simulink model "sim2_control_Architectures"  (R2022a)
settings: Solver=FixedStepAuto  StartTime=0.0  StopTime=8  FixedStep=0.001  RelTol=1e-3
undefined symbols (not defined in the file): a, b, c, DiscIntNeverNeededParam, k1, k2, kd2, kd3, kd4, ki3, kp1, kp2, kp3, kp4
libraries: slpidlib x2
settings Model: Creator=sokserey  LastModifiedBy=LabPC
settings DebuggingCC: UnconnectedInputMsg=warning  UnconnectedOutputMsg=warning  UnconnectedLineMsg=warning
settings RTWCC: DLArmComputeVersion=19.05

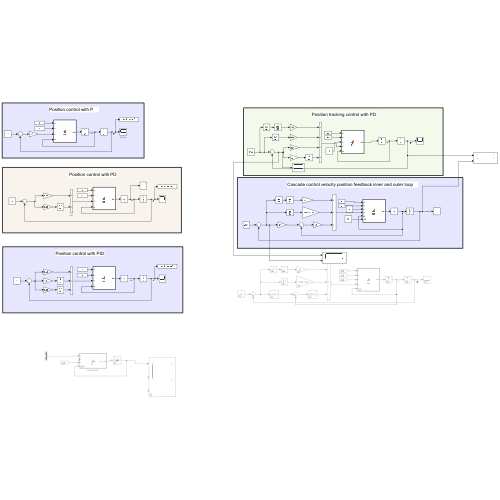
[thumbnail: Simulink's stored preview of the top-level diagram]
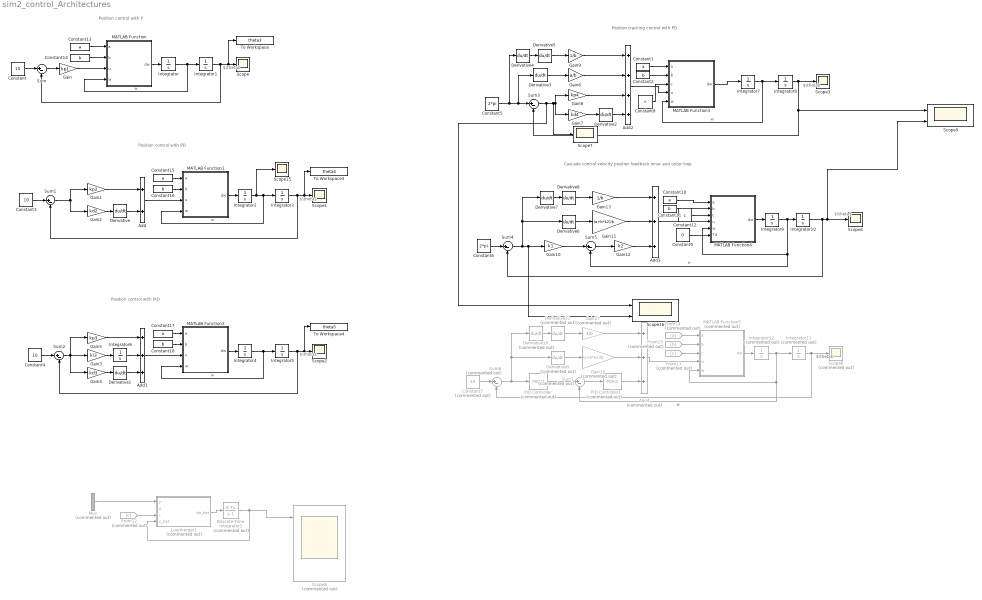
== system sim2_control_Architectures ==
  note: Position control with P
  note: Position control with PD
  note: $\theta$
  note: $\theta$
  note: $\theta$
  note: Position control with PID
  note: $\theta$
  note: Position tracking control with PD
  note: $\theta$
  note: Cascade control velocity position feedback inner and outer loop
  note: $\theta$
  Add : Sum
  Add1 : Sum  Inputs=+++
  Add2 : Sum  Inputs=++++
  Add3 : Sum  Inputs=+++
  Add4 : Sum  Commented=on  Inputs=+++
  Constant : Constant  Value=10
  Constant{1,10,13,15,17} (5 alike) : Constant  Value=a
  Constant{2,11,14,16,18} (5 alike) : Constant  Value=b
  Constant12 : Constant  Value=c
  Constant3 : Constant  Value=10
  Constant4 : Constant  Value=10
  Constant5 : Constant  Value=2*pi
  Constant6 : Constant  Value=2*pi
  Constant7 : Constant  Commented=on  Value=10
  Constant8 : Constant  Value=c
  Constant9 : Constant  Value=0
  Derivative{,1..8} (9 alike) : Derivative
  Derivative10 : Derivative  Commented=on
  Derivative11 : Derivative  Commented=on
  Derivative9 : Derivative  Commented=on
  Discrete-Time Integrator2 : DiscreteIntegrator  Commented=on  InitialCondition=[0;0]  SampleTime=0.01  ICPrevOutput=DiscIntNeverNeededParam  ICPrevScaledInput=DiscIntNeverNeededParam
  From12 : From  Commented=on  GotoTag=c
  From13 : From  Commented=on  GotoTag=c
  From14 : From  Commented=on  GotoTag=a
  From15 : From  Commented=on  GotoTag=b
  Gain : Gain  Gain=kp1
  Gain1 : Gain  Gain=kp2
  Gain10 : Gain  Gain=k1
  Gain11 : Gain  Gain=(a+b*k2)/b
  Gain12 : Gain  Gain=k2
  Gain13 : Gain  Gain=1/b
  Gain15 : Gain  Commented=on  Gain=(a+b*k2)/b
  Gain17 : Gain  Commented=on  Gain=1/b
  Gain2 : Gain  Gain=kd2
  Gain3 : Gain  Gain=ki3
  Gain4 : Gain  Gain=kd3
  Gain5 : Gain  Gain=kp3
  Gain6 : Gain  Gain=kp4
  Gain7 : Gain  Gain=kd4
  Gain8 : Gain  Gain=a/b
  Gain9 : Gain  Gain=1/b
  Integrator{,1..10} (11 alike) : Integrator
  Integrator11 : Integrator  Commented=on
  Integrator12 : Integrator  Commented=on
  Luenberger1 : MATLAB Function  Commented=on  TreatAsAtomicUnit=on
  MATLAB Function : MATLAB Function  TreatAsAtomicUnit=on
  MATLAB Function1 : MATLAB Function  TreatAsAtomicUnit=on
  MATLAB Function2 : MATLAB Function  TreatAsAtomicUnit=on
  MATLAB Function3 : MATLAB Function  TreatAsAtomicUnit=on
  MATLAB Function4 : MATLAB Function  TreatAsAtomicUnit=on
  MATLAB Function5 : MATLAB Function  Commented=on  TreatAsAtomicUnit=on
  Mux : Mux  Commented=on  Inputs=2
  PID Controller : slpidlib/PID Controller  Commented=on  Controller=PID  Form=Parallel  TimeDomain=Discrete-time  UseExternalTs=off  SampleTime=-1  IntegratorMethod=Forward Euler  FilterMethod=Forward Euler  ControllerParametersSource=internal  P=0.000211921225364968  I=9.98226441094489e-09  UseKiTs=off  D=0.999605299326111  N=0.722686382801031  UseFilter=on  TunerSelectOption=Transfer Function Based (PID Tuner App)  InitialConditionSource=internal  InitialConditionForIntegrator=0  InitialConditionForFilter=0  DifferentiatorICPrevScaledInput=0  ExternalReset=none  TrackingMode=off  Kt=1  LimitOutput=off  SatLimitsSource=internal  UpperSaturationLimit=inf  LowerSaturationLimit=-inf  LinearizeAsGain=on  AntiWindupMode=none  Kb=1  POutMin=[]  POutMax=[]  IOutMin=[]  IOutMax=[]  DOutMin=[]  DOutMax=[]  NOutMin=[]  NOutMax=[]  SumOutMin=[]  SumOutMax=[]  SaturationOutMin=[]  SaturationOutMax=[]  PParamMin=[]  PParamMax=[]  IParamMin=[]  IParamMax=[]  DParamMin=[]  DParamMax=[]  NParamMin=[]  NParamMax=[]  KbParamMin=[]  KbParamMax=[]  KtParamMin=[]  KtParamMax=[]  KbOutMin=[]  KbOutMax=[]  KtOutMin=[]  KtOutMax=[]  IntegratorOutMin=[]  IntegratorOutMax=[]  FilterOutMin=[]  FilterOutMax=[]  SumI1OutMin=[]  SumI1OutMax=[]  SumI2OutMin=[]  SumI2OutMax=[]  SumI3OutMin=[]  SumI3OutMax=[]  SumI4OutMin=[]  SumI4OutMax=[]  SumDOutMin=[]  SumDOutMax=[]  DifferentiatorOutMin=[]  DifferentiatorOutMax=[]  FilterDiffOutCoefMin=[]  FilterDiffOutCoefMax=[]  ReciprocalOutMin=[]  ReciprocalOutMax=[]  SumDenOutMin=[]  SumDenOutMax=[]  SumNumOutMin=[]  SumNumOutMax=[]  DivideOutMin=[]  DivideOutMax=[]  UdiffTsProdOutMin=[]  UdiffTsProdOutMax=[]  NTsProdOutMin=[]  NTsProdOutMax=[]  UintegralTsProdOutMin=[]  UintegralTsProdOutMax=[]  UngainTsProdOutMin=[]  UngainTsProdOutMax=[]  IntegratorContinuousStateAttributes=''  IntegratorStateMustResolveToSignalObject=off  IntegratorRTWStateStorageClass=Auto  FilterContinuousStateAttributes=''  FilterStateMustResolveToSignalObject=off  FilterRTWStateStorageClass=Auto  ParallelPVariant=InternalParameters  IdealPVariant=Disabled  IVariant=InternalParameters  DVariant=InternalParameters  IntegratorVariant=Discrete  SatVariant=Disabled  AWVariant=Passthrough  PCopyVariant=Disabled  TRVariant=Disabled  FdbkBlocksVariant=Forward  IdealPFdbkVariant=Disabled  SatFdbkVariant=Disabled  DerivativeFilterVariant=ForwardEulerFilter  NVariant=InternalParameters  NCopyVariant=Disabled  FilterICVariant=InternalICsFilter  IntegratorICVariant=InternalICs  ExternalResetVariant=Disabled  TRSumVariant=Passthrough  SumFdbkVariant=Disabled  SumVariant=Sum_PID  TsampFilterVariant=InternalTs  TsampNgainVariant=Passthrough  TsampIntegralVariant=Passthrough  ExternalSaturationOutDataTypeStr=Inherit: Same as second input  aMode=0
  PID Controller1 : slpidlib/PID Controller  Commented=on  Controller=PID  Form=Parallel  TimeDomain=Discrete-time  UseExternalTs=off  SampleTime=-1  IntegratorMethod=Forward Euler  FilterMethod=Forward Euler  ControllerParametersSource=internal  P=0.27  I=1  UseKiTs=off  D=0  N=100  UseFilter=on  TunerSelectOption=Transfer Function Based (PID Tuner App)  InitialConditionSource=internal  InitialConditionForIntegrator=0  InitialConditionForFilter=0  DifferentiatorICPrevScaledInput=0  ExternalReset=none  TrackingMode=off  Kt=1  LimitOutput=off  SatLimitsSource=internal  UpperSaturationLimit=inf  LowerSaturationLimit=-inf  LinearizeAsGain=on  AntiWindupMode=none  Kb=1  POutMin=[]  POutMax=[]  IOutMin=[]  IOutMax=[]  DOutMin=[]  DOutMax=[]  NOutMin=[]  NOutMax=[]  SumOutMin=[]  SumOutMax=[]  SaturationOutMin=[]  SaturationOutMax=[]  PParamMin=[]  PParamMax=[]  IParamMin=[]  IParamMax=[]  DParamMin=[]  DParamMax=[]  NParamMin=[]  NParamMax=[]  KbParamMin=[]  KbParamMax=[]  KtParamMin=[]  KtParamMax=[]  KbOutMin=[]  KbOutMax=[]  KtOutMin=[]  KtOutMax=[]  IntegratorOutMin=[]  IntegratorOutMax=[]  FilterOutMin=[]  FilterOutMax=[]  SumI1OutMin=[]  SumI1OutMax=[]  SumI2OutMin=[]  SumI2OutMax=[]  SumI3OutMin=[]  SumI3OutMax=[]  SumI4OutMin=[]  SumI4OutMax=[]  SumDOutMin=[]  SumDOutMax=[]  DifferentiatorOutMin=[]  DifferentiatorOutMax=[]  FilterDiffOutCoefMin=[]  FilterDiffOutCoefMax=[]  ReciprocalOutMin=[]  ReciprocalOutMax=[]  SumDenOutMin=[]  SumDenOutMax=[]  SumNumOutMin=[]  SumNumOutMax=[]  DivideOutMin=[]  DivideOutMax=[]  UdiffTsProdOutMin=[]  UdiffTsProdOutMax=[]  NTsProdOutMin=[]  NTsProdOutMax=[]  UintegralTsProdOutMin=[]  UintegralTsProdOutMax=[]  UngainTsProdOutMin=[]  UngainTsProdOutMax=[]  IntegratorContinuousStateAttributes=''  IntegratorStateMustResolveToSignalObject=off  IntegratorRTWStateStorageClass=Auto  FilterContinuousStateAttributes=''  FilterStateMustResolveToSignalObject=off  FilterRTWStateStorageClass=Auto  ParallelPVariant=InternalParameters  IdealPVariant=Disabled  IVariant=InternalParameters  DVariant=InternalParameters  IntegratorVariant=Discrete  SatVariant=Disabled  AWVariant=Passthrough  PCopyVariant=Disabled  TRVariant=Disabled  FdbkBlocksVariant=Forward  IdealPFdbkVariant=Disabled  SatFdbkVariant=Disabled  DerivativeFilterVariant=ForwardEulerFilter  NVariant=InternalParameters  NCopyVariant=Disabled  FilterICVariant=InternalICsFilter  IntegratorICVariant=InternalICs  ExternalResetVariant=Disabled  TRSumVariant=Passthrough  SumFdbkVariant=Disabled  SumVariant=Sum_PID  TsampFilterVariant=InternalTs  TsampNgainVariant=Passthrough  TsampIntegralVariant=Passthrough  ExternalSaturationOutDataTypeStr=Inherit: Same as second input  aMode=0
  Scope{,1..4,7,15} (7 alike) : Scope
  Scope16 : Scope  NumInputPorts=2
  Scope5 : Scope  NumInputPorts=2
  Scope6 : Scope  Commented=on
  Scope8 : Scope  Commented=on  NumInputPorts=3
  Sum{,1..5} (6 alike) : Sum  Inputs=|+-
  Sum6 : Sum  Commented=on  Inputs=|+-
  Sum7 : Sum  Commented=on  Inputs=|+-
  To Workspace : ToWorkspace  VariableName=theta3  SampleTime=-1
      settings: Save2DSignal=2-D array (concatenate along first dimension)
  To Workspace3 : ToWorkspace  VariableName=theta4  SampleTime=-1
      settings: Save2DSignal=2-D array (concatenate along first dimension)
  To Workspace4 : ToWorkspace  VariableName=theta5  SampleTime=-1
      settings: Save2DSignal=2-D array (concatenate along first dimension)
  wires:
  Gain/1 -> MATLAB Function/3(u)
  Sum2/1 -> Gain4/1, Gain5/1, Gain3/1
  Constant16/1 -> MATLAB Function1/2(b)
  Add1/1 -> MATLAB Function2/3(u)
  Integrator1/1 -> Sum/2, To Workspace/1, Scope/1
  Sum/1 -> Gain/1
  Gain5/1 -> Add1/1
  Constant4/1 -> Sum2/1
  Gain1/1 -> Add/1
  MATLAB Function2/1(dw) -> Integrator4/1
  Constant15/1 -> MATLAB Function1/1(a)
  Constant3/1 -> Sum1/1
  Gain4/1 -> Derivative1/1
  Derivative/1 -> Add/2
  Integrator5/1 -> Sum2/2, Scope2/1, To Workspace4/1
  Add/1 -> MATLAB Function1/3(u)
  Integrator2/1 -> Scope15/1, MATLAB Function1/4(w), Integrator3/1  "w"
  Integrator/1 -> Integrator1/1, MATLAB Function/4(w)  "w"
  Integrator4/1 -> Integrator5/1, MATLAB Function2/4(w)  "w"
  Constant18/1 -> MATLAB Function2/2(b)
  Sum1/1 -> Gain2/1, Gain1/1
  Constant17/1 -> MATLAB Function2/1(a)
  Gain2/1 -> Derivative/1
  Gain3/1 -> Integrator6/1
  Integrator3/1 -> To Workspace3/1, Scope1/1, Sum1/2
  Constant/1 -> Sum/1
  MATLAB Function/1(dw) -> Integrator/1
  Derivative1/1 -> Add1/3
  MATLAB Function1/1(dw) -> Integrator2/1
  Integrator6/1 -> Add1/2
  Integrator8/1 -> Scope5/1, Sum3/2, Scope3/1
  Gain7/1 -> Derivative2/1
  Sum3/1 -> Scope16/1, Scope7/1, Gain6/1, Gain7/1
  Integrator7/1 -> Integrator8/1, MATLAB Function3/5(w)  "w"
  Add2/1 -> MATLAB Function3/4(u)
  Constant5/1 -> Derivative4/1, Derivative3/1, Sum3/1
  Constant1/1 -> MATLAB Function3/1(a)
  Constant2/1 -> MATLAB Function3/2(b)
  Gain9/1 -> Add2/1
  Gain8/1 -> Add2/2
  Gain6/1 -> Add2/3
  Derivative2/1 -> Add2/4
  MATLAB Function3/1(dw) -> Integrator7/1
  Derivative3/1 -> Gain8/1
  Derivative4/1 -> Derivative5/1
  Derivative5/1 -> Gain9/1
  MATLAB Function4/1(dw) -> Integrator9/1
  Integrator10/1 -> Scope5/2, Scope4/1, Sum4/2
  Sum4/1 -> Derivative6/1, Derivative7/1, Scope16/2, Gain10/1
  Integrator9/1 -> Integrator10/1, MATLAB Function4/5(w), Sum5/2  "w"
  Constant6/1 -> Sum4/1
  Gain10/1 -> Sum5/1
  Sum5/1 -> Gain12/1
  Gain12/1 -> Add3/3
  Gain11/1 -> Add3/2
  Gain13/1 -> Add3/1
  Derivative7/1 -> Derivative8/1
  Derivative8/1 -> Gain13/1
  Derivative6/1 -> Gain11/1
  Add3/1 -> MATLAB Function4/4(u)
  Constant8/1 -> MATLAB Function3/3(c)
  Luenberger1/1(dx_hat) -> Discrete-Time Integrator2/1
  Discrete-Time Integrator2/1 -> Luenberger1/4(x_hat), Scope8/1
  Mux/1 -> Luenberger1/1(y)
  From12/1 -> Luenberger1/3(c)
  From13/1 -> MATLAB Function5/3(c)
  Add4/1 -> MATLAB Function5/4(u)
  Derivative9/1 -> Gain15/1
  Derivative11/1 -> Gain17/1
  Derivative10/1 -> Derivative11/1
  Gain17/1 -> Add4/1
  Gain15/1 -> Add4/2
  PID Controller1/1 -> Add4/3
  Sum7/1 -> PID Controller1/1
  PID Controller/1 -> Sum7/1
  From15/1 -> MATLAB Function5/2(b)
  From14/1 -> MATLAB Function5/1(a)
  Constant7/1 -> Sum6/1
  Integrator12/1 -> Integrator11/1, Sum7/2, MATLAB Function5/5(w)  "w"
  Sum6/1 -> PID Controller/1, Derivative10/1, Derivative9/1
  Integrator11/1 -> Sum6/2, Scope6/1
  MATLAB Function5/1(dw) -> Integrator12/1
  Constant9/1 -> MATLAB Function4/6(Td)
  Constant10/1 -> MATLAB Function4/1(a)
  Constant11/1 -> MATLAB Function4/2(b)
  Constant12/1 -> MATLAB Function4/3(c)
  Constant13/1 -> MATLAB Function/1(a)
  Constant14/1 -> MATLAB Function/2(b)

== matlab function sim2_control_Architectures/MATLAB Function3 ==
  data: a input; dw output; b input; c input; u input; w input
function dw = fcn(a,b,c,u,w)

dw = -a*w+b*u-c*sign(w);

== matlab function sim2_control_Architectures/MATLAB Function4 ==
  data: a input; dw output; b input; c input; u input; w input; Td input
function dw = fcn(a,b,c,u,w,Td)

dw = -a*w+b*u-c*sign(w)+Td;

== matlab function sim2_control_Architectures/MATLAB Function5 ==
  data: a input; dw output; b input; c input; u input; w input
function dw = fcn(a,b,c,u,w)

dw = -a*w+b*u-c*sign(w);

== matlab function sim2_control_Architectures/MATLAB Function ==
  data: a input; dw output; b input; u input; w input
function dw = fcn(a,b,u,w)

dw = -a*w+b*u;

== matlab function sim2_control_Architectures/MATLAB Function1 ==
  data: a input; dw output; b input; u input; w input
function dw = fcn(a,b,u,w)

dw = -a*w+b*u;

== matlab function sim2_control_Architectures/MATLAB Function2 ==
  data: a input; dw output; b input; u input; w input
function dw = fcn(a,b,u,w)

dw = -a*w+b*u;

== matlab function sim2_control_Architectures/Luenberger1 ==
  data: y input; u input; c input; dx_hat output; x_hat input
function dx_hat = fcn(y,u,c,x_hat)

Ke=[1;10];
a=26.85;
b=85.68;
A = [-a 0;1 0];
B = [b;0];
C = [0 1];
dx_hat = A*x_hat + B*u +c*sign(x_hat(1,1)) + Ke.*(y - C*x_hat);
